simulink model "SerialReceive"  (R2015b)
settings: Solver=VariableStepAuto  StartTime=0.0  StopTime=10.0  RelTol=1e-3
undefined symbols (not defined in the file or in its folder): LF, serial
libraries: instrumentlib x2, xpcseriallib x1
settings Model: Creator=TOOsab  LastModifiedBy=TOOsab

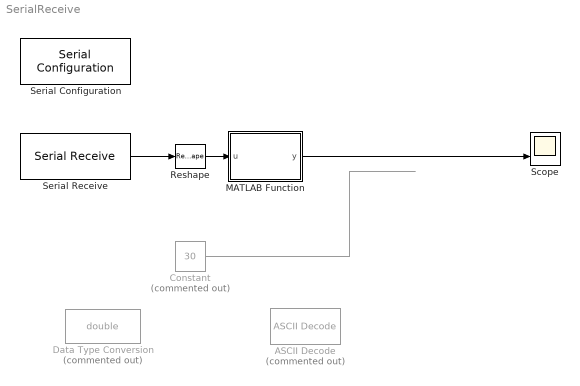
== system SerialReceive ==
  "ASCII Decode " : xpcseriallib/ASCII Decode   Commented=on  format=%u\n  nvars=1  vartypes={ }
  Constant : Constant  Commented=on  Value=30
  Data Type Conversion : DataTypeConversion  Commented=on  OutDataTypeStr=double
  MATLAB Function : MATLAB Function  TreatAsAtomicUnit=on
  Reshape : Reshape  OutputDimensionality=Customize  OutputDimensions=[1]
  Scope : Scope  NumInputPorts=2
  Serial Configuration : instrumentlib/Serial Configuration  Priority=-200000  ComPortMenu=COM4  ComPort=COM4  ObjConstructor=serial('COM4');  BaudRate=115200  DataBits=8  Parity=none  StopBits=1  FlowControl=none  Timeout=10  ByteOrder=LittleEndian
  Serial Receive : instrumentlib/Serial Receive  ComPortMenu=COM4  ComPort=COM4  ObjConstructor=serial('COM4');  Terminator=LF ('\n')  DataSize="[1  1]"  DataType=int8  EnableBlockingMode=on  ActionDataUnavailable=Output last received value  CustomValue=0  SampleTime=0.01
  wires:
  Constant/1 -> ?
  Serial Receive/1 -> Reshape/1
  MATLAB Function/1(y) -> Scope/2
  Reshape/1 -> MATLAB Function/1(u)

== matlab function SerialReceive/MATLAB Function ==
  data: u input; y output
function y = fcn(u)
%#codegen
g = eye(3);
%y=1;
y = unicode2native(u);
